simulink model "udp_send"  (R2016b)
settings: Solver=VariableStepAuto  StartTime=0.0  StopTime=inf  RelTol=1e-3
libraries: xpcrtudplib x1
settings Model: Creator=zeabus  LastModifiedBy=zeabus

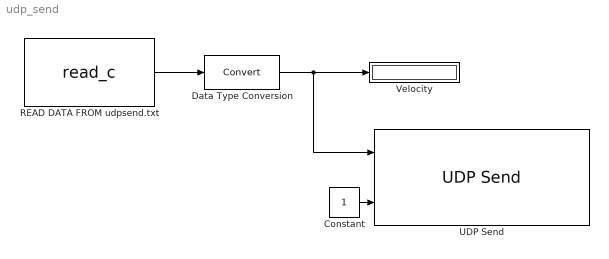
== system udp_send ==
  Constant : Constant
  Data Type Conversion : DataTypeConversion
  READ DATA FROM udpsend.txt : S-Function  FunctionName=read_c  SFunctionModules='read_c'  SFunctionDeploymentMode=off  EnableBusSupport=off
  UDP Send : xpcrtudplib/UDP Send  ipAddressVal=Use host-target connection  localPort=25001  toAddress=10.213.150.118  toPort=20002  sampleTime=0.01
  Velocity : Display
  wires:
  READ DATA FROM udpsend.txt/1 -> Data Type Conversion/1
  Data Type Conversion/1 -> UDP Send/1, Velocity/1
  Constant/1 -> UDP Send/2
